simulink model "SequenceSeparation_Debug"  (R2018a)
settings: Solver=ode5  StartTime=0.0  StopTime=0.2  FixedStep=Ts  RelTol=1e-3
InitFcn:
  | SequenceSeparation_script
values from neighbouring files (symbols this model uses):
  Fn = 50    [SequenceSeparation_script.m]
  Lr = Vdc / (0.8 * 2^0.5 * ( Sn / 3^0.5 / Vrms) * Fsw)    (= 0.001)    [SequenceSeparation_script.m]
  Rr = 0.005    [SequenceSeparation_script.m]
  Ts = 1e-6    (= 1e-06)    [SequenceSeparation_script.m]
  Ts_cont = 1/10000    (= 0.0001)    [SequenceSeparation_script.m]
  Ts_pwm = 1/200000    (= 5e-06)    [SequenceSeparation_script.m]
  Vdc = 2    [SequenceSeparation_script.m]
libraries: powerlib x12, pwrsysVSrc_202301 x2, pwrsysBasic_202301 x2, pwrsysVICtrl_202301 x1, pwrsysTransf_202301 x1
settings Model: Creator=daniemot  LastModifiedBy=daniemot

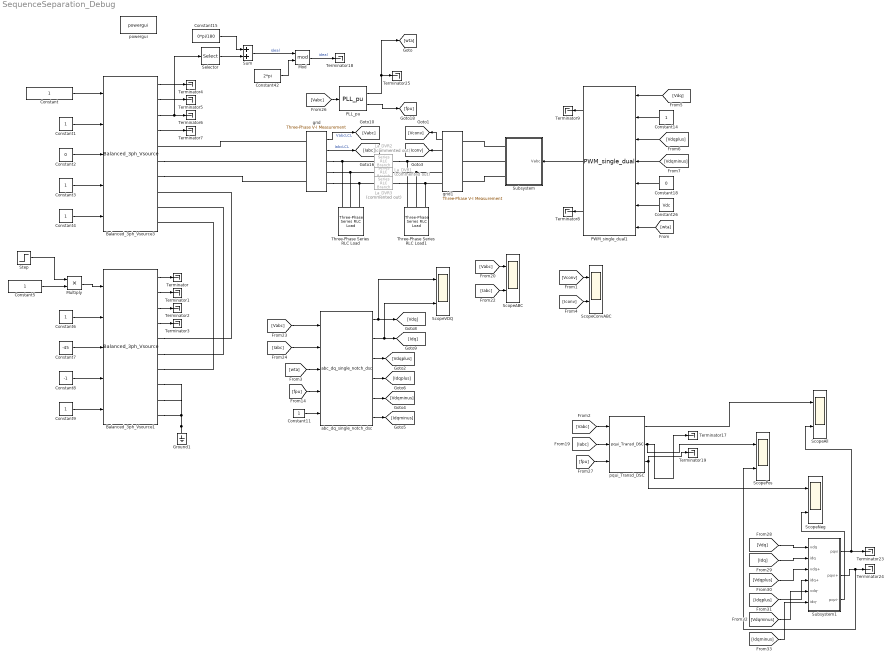
== system SequenceSeparation_Debug ==
  Balanced_3ph_Vsource1 : pwrsysVSrc_202301/Balanced_3ph_Vsource  BaseAmp=1  fn=50  AmpIni=1  SeqIni=1  AngIni=0  FIni=50  HarmIni=1
  Balanced_3ph_Vsource3 : pwrsysVSrc_202301/Balanced_3ph_Vsource  BaseAmp=1  fn=50  AmpIni=1  SeqIni=1  AngIni=0  FIni=50  HarmIni=1
  Constant{,1,3..6,9,11,14} (9 alike) : Constant
  Constant15 : Constant  Value=0*pi/180
  Constant18 : Constant  Value=0
  Constant2 : Constant  Value=0
  Constant26 : Constant  Value=Vdc
  Constant42 : Constant  Value=2*pi
  Constant7 : Constant  Value=-45
  Constant8 : Constant  Value=-1
  Ground1 : powerlib/Elements/Ground  LConnTagsString=a
  La_DVR1 : powerlib/Elements/Series RLC Branch  Commented=on  LConnTagsString=__new0  RConnTagsString=__new0  BranchType=RL  Resistance=Rr  Inductance=Lr  SetiL0=off  InitialCurrent=0  Capacitance=1.0  Setx0=off  InitialVoltage=0  Measurements=None
  La_DVR2 : powerlib/Elements/Series RLC Branch  Commented=on  LConnTagsString=__new0  RConnTagsString=__new0  BranchType=RL  Resistance=Rr  Inductance=Lr  SetiL0=off  InitialCurrent=0  Capacitance=1.0  Setx0=off  InitialVoltage=0  Measurements=None
  La_DVR3 : powerlib/Elements/Series RLC Branch  Commented=on  LConnTagsString=__new0  RConnTagsString=__new0  BranchType=RL  Resistance=Rr  Inductance=Lr  SetiL0=off  InitialCurrent=0  Capacitance=1.0  Setx0=off  InitialVoltage=0  Measurements=None
  Mod : Math  Operator=mod  SaturateOnIntegerOverflow=on
  Multiply : Product
  PLL_pu : pwrsysBasic_202301/PLL_pu  fn=Fn  Ts=Ts_cont  Kp_pll=90  Ki_pll=1600  Kd_pll=0  PLL_ini=30
  PWM_single_dual1 : pwrsysVICtrl_202301/PWM_single_dual  fsw=Fsw  Ts=Ts_pwm  Uabp=Vampline  PWM_Ini_Phase=90
  ScopeABC : Scope  NumInputPorts=2
  ScopeAll : Scope  NumInputPorts=2
  ScopeConvABC : Scope  NumInputPorts=2
  ScopeNeg : Scope  NumInputPorts=2
  ScopePos : Scope  NumInputPorts=2
  ScopeVDQ : Scope  NumInputPorts=2
  Selector : Selector  InputPortWidth=3  IndexOptions=Index vector (dialog)  Indices=[1]  OutputSizes=1
  Step : Step  Time=0.1  SampleTime=0
  Subsystem : Subsystem
  Subsystem1 : Subsystem
  Sum : Sum
  Terminator{,1..9,17..19,23..25} (16 alike) : Terminator
  Three-Phase Series RLC Load : powerlib/Elements/Three-Phase Series RLC Load  LConnTagsString=A|B|C  Configuration=Y (grounded)  NominalVoltage=(3/2)^0.5  Vabc=[1e3 1e3 1e3]  Vabcp=[1e3 1e3 1e3]  NominalFrequency=50  UnbalancedPower=off  ActivePower=0.01  InductivePower=0  CapacitivePower=0  Pabc=[10e3 9e3 11e3]  QLabc=[100 90 110]  QCabc=[100 90 110]  Pabcp=[10e3 9e3 11e3]  QLabcp=[100 90 110]  QCabcp=[100 90 110]  Measurements=None  LoadType=constant Z
  Three-Phase Series RLC Load1 : powerlib/Elements/Three-Phase Series RLC Load  LConnTagsString=A|B|C  Configuration=Y (grounded)  NominalVoltage=(3/2)^0.5  Vabc=[1e3 1e3 1e3]  Vabcp=[1e3 1e3 1e3]  NominalFrequency=50  UnbalancedPower=off  ActivePower=0.01  InductivePower=0  CapacitivePower=0  Pabc=[10e3 9e3 11e3]  QLabc=[100 90 110]  QCabc=[100 90 110]  Pabcp=[10e3 9e3 11e3]  QLabcp=[100 90 110]  QCabcp=[100 90 110]  Measurements=None  LoadType=constant Z
  abc_dq_single_notch_dsc : pwrsysTransf_202301/abc_dq_single_notch_dsc  Ts=Ts_cont  fn=2*Fn  zeta=0.707
  grid : powerlib/Measurements/Three-Phase V-I Measurement  VoltageMeasurement=phase-to-ground  SetLabelV=off  LabelV=vgrid  Vpu=off  VpuLL=off  CurrentMeasurement=yes  SetLabelI=off  LabelI=igrid  Ipu=off  Pbase=sn  Vbase=uab  OutputType=Complex  PhasorSimulation=off  PSBequivalent=0
  grid1 : powerlib/Measurements/Three-Phase V-I Measurement  VoltageMeasurement=phase-to-ground  SetLabelV=off  LabelV=vgrid  Vpu=off  VpuLL=off  CurrentMeasurement=yes  SetLabelI=off  LabelI=igrid  Ipu=off  Pbase=sn  Vbase=uab  OutputType=Complex  PhasorSimulation=off  PSBequivalent=0
  powergui : powerlib/powergui  Priority=1  SimulationMode=Discrete  SampleTime=Ts  frequency=60  Iterations=50  frequencyindice=0  Pbase=100e6  ErrMax=1e-4  UnitsV=kV  UnitsW=MW  buscounter=0  FunctionMessages=off  echomessages=off  EnableUseOfTLC=off  CurrentSourceSwitches=off  DisableSnubberDevices=off  DisableRonSwitches=off  DisableVfSwitches=off  DisplayEquations=off  SolverType=Tustin/Backward Euler (TBE)  Interpol=off  ExternalGateDelay=off  methode=off  Ts=100  x0status=blocks  SPID=off  SwTol=0  HookPort=off  RestoreLinks=warning  ResistiveCurrentMeasurement=off  Frange=[60:1:1600]  Ylog=on  Xlog=on  ShowGrid=on  save=off  variable=ZData  structure=0  ZoomFFT=off  StartTime=0.0  cycles=1  DisplayStyle=1  fundamental=60  FreqAxis=off  MaxFrequency=1000  frequencyindicesteady=1  RmsSteady=1  display=off
  pqui_Transd_DSC : pwrsysBasic_202301/pqui_Transd_DSC  Ts=Ts_cont  fn=Fn  Sn=1.5  Uanp=1  Iap=1
  wires:
  Constant/1 -> Balanced_3ph_Vsource3/1
  Constant1/1 -> Balanced_3ph_Vsource3/2
  Constant2/1 -> Balanced_3ph_Vsource3/3
  Constant3/1 -> Balanced_3ph_Vsource3/4
  Constant4/1 -> Balanced_3ph_Vsource3/5
  Constant8/1 -> Balanced_3ph_Vsource1/4
  Constant5/1 -> Multiply/2
  Constant9/1 -> Balanced_3ph_Vsource1/5
  Constant6/1 -> Balanced_3ph_Vsource1/2
  Constant7/1 -> Balanced_3ph_Vsource1/3
  Balanced_3ph_Vsource1/1 -> Terminator/1
  Balanced_3ph_Vsource1/2 -> Terminator1/1
  Balanced_3ph_Vsource1/3 -> Terminator2/1
  Balanced_3ph_Vsource1/4 -> Terminator3/1
  Balanced_3ph_Vsource3/1 -> Terminator4/1
  Balanced_3ph_Vsource3/4 -> Terminator7/1
  Balanced_3ph_Vsource3/2 -> Terminator5/1
  Balanced_3ph_Vsource3/3 -> Selector/1, Terminator6/1
  Selector/1 -> Sum/2
  Constant15/1 -> Sum/1
  Constant11/1 -> abc_dq_single_notch_dsc/5
  [wta] -> abc_dq_single_notch_dsc/3
  [fpu] -> abc_dq_single_notch_dsc/4
  grid/1 -> [Vabc]  "VabcLCL"
  Multiply/1 -> Balanced_3ph_Vsource1/1
  Step/1 -> Multiply/1
  abc_dq_single_notch_dsc/3 -> [Vdqplus]
  abc_dq_single_notch_dsc/5 -> [Vdqminus]
  abc_dq_single_notch_dsc/4 -> [Idqplus]
  abc_dq_single_notch_dsc/1 -> ScopeVDQ/1, [Vdq]
  abc_dq_single_notch_dsc/2 -> ScopeVDQ/2, [Idq]
  Sum/1 -> Mod/1  "ideal"
  Constant42/1 -> Mod/2
  grid/2 -> [Iabc]  "IabcLCL"
  [Vabc] -> abc_dq_single_notch_dsc/1
  [Iabc] -> abc_dq_single_notch_dsc/2
  [fpu] -> pqui_Transd_DSC/3
  [Vabc] -> pqui_Transd_DSC/1
  [Iabc] -> pqui_Transd_DSC/2
  [Vabc] -> PLL_pu/1
  PLL_pu/1 -> [wta], Terminator25/1
  PLL_pu/2 -> [fpu]
  Mod/1 -> Terminator18/1  "ideal"
  [Vdq] -> Subsystem1/1(vdq)
  [Idq] -> Subsystem1/2(idq)
  [Vdqplus] -> Subsystem1/3(vdq+)
  [Idqplus] -> Subsystem1/4(idq+)
  [Vdqminus] -> Subsystem1/5(vdq-)
  [Idqminus] -> Subsystem1/6(idq-)
  pqui_Transd_DSC/2 -> ScopePos/1, Terminator17/1
  pqui_Transd_DSC/3 -> ScopeNeg/1, Terminator19/1
  Subsystem1/1(pqvi) -> ScopeAll/2, Terminator23/1
  Subsystem1/2(pqvi+) -> ScopePos/2, Terminator24/1
  pqui_Transd_DSC/1 -> ScopeAll/1
  Subsystem1/3(pqvi-) -> ScopeNeg/2
  [Vabc] -> ScopeABC/1
  [Iabc] -> ScopeABC/2
  abc_dq_single_notch_dsc/6 -> [Idqminus]
  PWM_single_dual1/2 -> Subsystem/1(Vabc)
  Constant18/1 -> PWM_single_dual1/5
  PWM_single_dual1/3 -> Terminator8/1
  Constant14/1 -> PWM_single_dual1/2
  Constant26/1 -> PWM_single_dual1/6
  [wta] -> PWM_single_dual1/7
  PWM_single_dual1/1 -> Terminator9/1
  [Vdq] -> PWM_single_dual1/1
  [Vdqplus] -> PWM_single_dual1/3
  [Vdqminus] -> PWM_single_dual1/4
  grid1/1 -> [Vconv]
  grid1/2 -> [Iconv]
  [Vconv] -> ScopeConvABC/1
  [Iconv] -> ScopeConvABC/2
  connections:
  Ground1/LConn1 -- Balanced_3ph_Vsource1/RConn6 -- Balanced_3ph_Vsource1/RConn5 -- Balanced_3ph_Vsource1/RConn4
  Balanced_3ph_Vsource1/RConn3 -- Balanced_3ph_Vsource3/RConn6
  Balanced_3ph_Vsource1/RConn2 -- Balanced_3ph_Vsource3/RConn5
  Balanced_3ph_Vsource1/RConn1 -- Balanced_3ph_Vsource3/RConn4
  grid/LConn1 -- Balanced_3ph_Vsource3/RConn1
  Balanced_3ph_Vsource3/RConn2 -- grid/LConn2
  Balanced_3ph_Vsource3/RConn3 -- grid/LConn3
  Subsystem/RConn1 -- grid1/LConn1
  Subsystem/RConn3 -- grid1/LConn3
  Subsystem/RConn2 -- grid1/LConn2
  grid/RConn1 -- La_DVR2/RConn1 -- Three-Phase Series RLC Load/LConn1
  grid/RConn2 -- La_DVR1/RConn1 -- Three-Phase Series RLC Load/LConn2
  grid/RConn3 -- La_DVR3/RConn1 -- Three-Phase Series RLC Load/LConn3
  grid1/RConn1 -- La_DVR2/LConn1 -- Three-Phase Series RLC Load1/LConn1
  grid1/RConn2 -- La_DVR1/LConn1 -- Three-Phase Series RLC Load1/LConn2
  grid1/RConn3 -- La_DVR3/LConn1 -- Three-Phase Series RLC Load1/LConn3

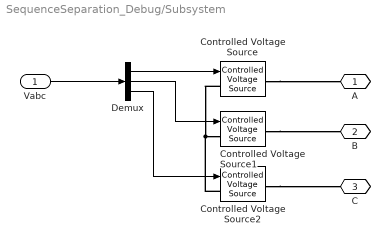
== system SequenceSeparation_Debug/Subsystem ==
  Vabc : Inport
  Controlled Voltage Source : powerlib/Electrical Sources/Controlled Voltage Source  Initialize=off  Source_Type=DC  Amplitude=0  Phase=0  Frequency=0  Measurements=None
  Controlled Voltage Source1 : powerlib/Electrical Sources/Controlled Voltage Source  Initialize=off  Source_Type=DC  Amplitude=0  Phase=0  Frequency=0  Measurements=None
  Controlled Voltage Source2 : powerlib/Electrical Sources/Controlled Voltage Source  Initialize=off  Source_Type=DC  Amplitude=0  Phase=0  Frequency=0  Measurements=None
  Demux : Demux  Outputs=3
  A : PMIOPort  Side=Right
  B : PMIOPort  Port=2  Side=Right
  C : PMIOPort  Port=3  Side=Right
  wires:
  Vabc/1 -> Demux/1
  Demux/2 -> Controlled Voltage Source1/1
  Demux/1 -> Controlled Voltage Source/1
  Demux/3 -> Controlled Voltage Source2/1
  connections:
  Controlled Voltage Source/LConn1 -- Controlled Voltage Source2/LConn1 -- Controlled Voltage Source1/LConn1
  Controlled Voltage Source1/RConn1 -- B/RConn1
  Controlled Voltage Source2/RConn1 -- C/RConn1
  Controlled Voltage Source/RConn1 -- A/RConn1

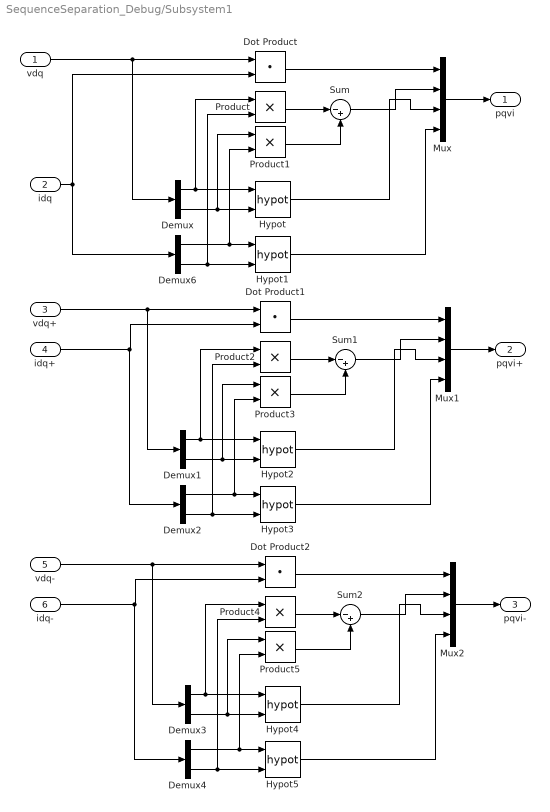
== system SequenceSeparation_Debug/Subsystem1 ==
  vdq : Inport
  idq : Inport  Port=2
  vdq+ : Inport  Port=3
  idq+ : Inport  Port=4
  vdq- : Inport  Port=5
  idq- : Inport  Port=6
  Demux{,1..4,6} (6 alike) : Demux  Outputs=2
  Dot Product : DotProduct  InputSameDT=on  OutDataTypeStr=Inherit: Inherit via internal rule
  Dot Product1 : DotProduct  InputSameDT=on  OutDataTypeStr=Inherit: Inherit via internal rule
  Dot Product2 : DotProduct  InputSameDT=on  OutDataTypeStr=Inherit: Inherit via internal rule
  Hypot{,1..5} (6 alike) : Math  Operator=hypot  SaturateOnIntegerOverflow=on
  Mux : Mux
  Mux1 : Mux
  Mux2 : Mux
  Product{,1..5} (6 alike) : Product
  Sum : Sum  Inputs=|-+
  Sum1 : Sum  Inputs=|-+
  Sum2 : Sum  Inputs=|-+
  pqvi : Outport
  pqvi+ : Outport  Port=2
  pqvi- : Outport  Port=3
  wires:
  idq/1 -> Dot Product/2, Demux6/1
  vdq/1 -> Demux/1, Dot Product/1
  Demux/1 -> Product/1, Hypot/1
  Demux/2 -> Product1/1, Hypot/2
  Demux6/2 -> Product/2, Hypot1/2
  Demux6/1 -> Product1/2, Hypot1/1
  Product/1 -> Sum/1
  Product1/1 -> Sum/2
  Dot Product/1 -> Mux/1
  Sum/1 -> Mux/2
  Hypot/1 -> Mux/3
  Hypot1/1 -> Mux/4
  Mux/1 -> pqvi/1
  Demux2/2 -> Product2/2, Hypot3/2
  Dot Product1/1 -> Mux1/1
  Mux1/1 -> pqvi+/1
  Hypot2/1 -> Mux1/3
  Sum1/1 -> Mux1/2
  Hypot3/1 -> Mux1/4
  Demux1/2 -> Product3/1, Hypot2/2
  Product2/1 -> Sum1/1
  Demux1/1 -> Product2/1, Hypot2/1
  Demux2/1 -> Product3/2, Hypot3/1
  Product3/1 -> Sum1/2
  vdq+/1 -> Demux1/1, Dot Product1/1
  idq+/1 -> Demux2/1, Dot Product1/2
  Demux4/1 -> Product5/2, Hypot5/1
  Demux3/1 -> Product4/1, Hypot4/1
  Demux3/2 -> Product5/1, Hypot4/2
  Product4/1 -> Sum2/1
  Hypot5/1 -> Mux2/4
  Hypot4/1 -> Mux2/3
  Sum2/1 -> Mux2/2
  Dot Product2/1 -> Mux2/1
  Mux2/1 -> pqvi-/1
  Demux4/2 -> Product4/2, Hypot5/2
  vdq-/1 -> Demux3/1, Dot Product2/1
  idq-/1 -> Demux4/1, Dot Product2/2
  Product5/1 -> Sum2/2
